simulink model "Q5_Electrical_CKT"  (R2020b)
settings: Solver=VariableStepAuto  StartTime=0.0  StopTime=10  MaxStep=0.2  RelTol=1e-3
values from neighbouring files (symbols this model uses):
  c = 10.0    [data_dict.sldd]
  R = 10.0    [data_dict.sldd]
settings Model: DataDictionary=data_dict.sldd  Creator=Shree  LastModifiedBy=Shree

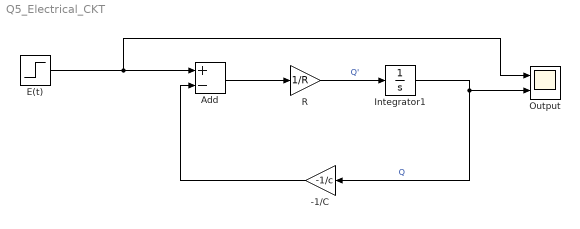
== system Q5_Electrical_CKT ==
  -1/C : Gain  Gain=-1/c
  Add : Sum  Inputs=+-
  E(t) : Step  SampleTime=0
  Integrator1 : Integrator  InitialCondition=1
  Output : Scope  NumInputPorts=2
  R : Gain  Gain=1/R
  wires:
  Add/1 -> R/1
  R/1 -> Integrator1/1  "Q'"
  -1/C/1 -> Add/2
  Integrator1/1 -> Output/2, -1/C/1  "Q"
  E(t)/1 -> Output/1, Add/1
